simulink model "ev_model_dc7"  (R2020a)
settings: Solver=FixedStepDiscrete  StartTime=0.0  StopTime=20  RelTol=1e-3  EnableMultiTasking=on
PreLoadFcn:
  | assignin('base','Ts',1e-6)
values from neighbouring files (symbols this model uses):
  m = ftell(file)    [calc_coeff.m]    (also in curve_fit_with_error_estimates.m = mean(cp); reheatTest.m = (h6-h5)/(h2-h5))
  s = [s12, s23, s34, s41]    [Rankine.m]    (also in annotation_ifelse.m = subplot(1,2,2); robotic_arm.m = [0]; test_otto.m = plot([0,l2*sind(theta)],             [0,l2*cosd(theta)],    )
undefined symbols (not defined in the file or in its folder): Ion, Lithium
libraries: electricdrivelib x2, powerlib x2, autolibshared x1
settings Model: ExtModeAutoUpdateStatusClock=off  Creator=MathWorks  LastModifiedBy=joshi
settings SolverCC: AutoInsertRateTranBlk=on
settings DataIOCC: LimitDataPoints=on  SaveFormat=Array  SignalLoggingSaveFormat=ModelDataLogs  SaveOutput=off  SignalLogging=off  SaveTime=off  ReturnWorkspaceOutputs=off  SignalLoggingName=sigsOut
settings OptimizationCC: ExpressionDepthLimit=2147483647  InitFltsAndDblsToZero=on  LifeSpan=inf
settings DebuggingCC: UnderspecifiedInitializationDetection=Classic  MergeDetectMultiDrivingBlocksExec=none  CheckExecutionContextPreStartOutputMsg=on  CheckExecutionContextRuntimeOutputMsg=on  SignalResolutionControl=TryResolveAllWithWarning  MultiTaskDSMMsg=warning  MultiTaskCondExecSysMsg=none  FcnCallInpInsideContextMsg=warning  StateNameClashWarn=warning  SFUnexpectedBacktrackingDiag=warning  SFNoUnconditionalDefaultTransitionDiag=warning  SFExecutionAtInitializationDiag=none  ArithmeticOperatorsInVariantConditions=warning
settings HardwareCC: ProdBitPerPointer=32  ProdBitPerSizeT=32  ProdBitPerPtrDiffT=32  ProdLargestAtomicFloat=None  ProdIntDivRoundTo=Undefined  ProdEndianess=Unspecified  ProdWordSize=32  ProdHWDeviceType=32-bit Generic  TargetUnknown=on
settings ModelReferenceCC: PropagateSignalLabelsOutOfModel=off
settings SFSimCC: SimUseLocalCustomCode=off  CustomCodeUndefinedFunction=UseInterfaceOnly
settings RTWCC: RTWUseLocalCustomCode=off
settings CodeAppCC: StateflowObjectComments=on
settings GRTTargetCC: TargetLangStandard=C89/C90 (ANSI)  CombineOutputUpdateFcns=off  GRTInterface=on
settings ConfigComp: CovMetricSettings=dw  CovHtmlReporting=on  CovSaveCumulativeToWorkspaceVar=on  CovSaveSingleToWorkspaceVar=on  CovExternalEMLEnable=off  CovSFcnEnable=off
settings SimscapeCC: SimscapeNormalizeSystem=off

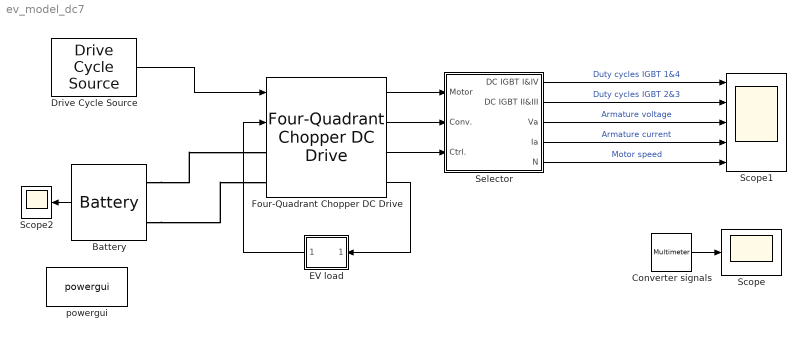
== system ev_model_dc7 ==
  Battery : electricdrivelib/Extra Sources/Battery  BatType=Lithium-Ion  ShowTempParam=off  ThermalPreset=no  ShowAgeParam=off  NomV=352  NomQ=120  SOC=100  Batt_Tr=2  PresetModel=on  MaxQ=120  MinV=264  FullV=409.7235  Dis_rate=52.1739  R=0.029333  Normal_OP=108.5217  expZone="[380.2958      5.895652]"  current=[6.5 13 32.5]  Units=Time  Tci=20  NomT=20  T2=-30  MaxQ2=4.8  FullV2=7.1  Normal_OP2=5.655  expZone2="[6.58           1]"  Rca=0.6  ti=2000  Dp=0  Neq0=0  Tsim=1e6  Ta1=25  Qeol=5.4*0.9  Reol=0.013333*1.2  Char_age=[2.3478, 3]  Dis_age=[2.3478, 10]  N1=1500  N2=10500  N3=1000  N4=1400  Ta2=45  N5=950
  Converter signals : powerlib/Measurements/Multimeter  PhasorSimulation=off  OutputType=Complex  sel=[5 6]  L=10  Gain=[1 1]  yselected={'Uab: Four-Quadrant Chopper DC Drive/Chopper/Chopper/Detailed_4q/IGBT//Diode','Udc: Four-Quadrant Chopper DC Drive/Chopper/Chopper/Detailed_4q/IGBT//Diode'};  PSBOutputType=1  PSBequivalent=0  AxesSetting=[0,0.1,-100,100]  Display=0  SavedBlockNames=-11
      settings: SourceProductBaseCode=MT,PS
  Drive Cycle Source : autolibshared/Drive Cycle Source  cycleVar=.mat, .xls, .xlsx or .txt file  fileVar=D:\MATLAb code files\drive_cycle_ev_dc7.xlsx  tfinal="20  seconds"  cycleRepeat=off  outAccPort=off  outGearPort=off  gearList=No gear data  t_wot1=5  xdot_woto=0  xdot_wot1=30  t_wot2=20  xdot_wot2=0  t_wotend=30  srcUnit=m/s  outUnit=m/s  srcAccUnit=m/s/s  outAccUnit=m/s^2  dt=0.5  aMode=1  faultOption=off  velBnd=2  velBndUnit=mph  inUnit=m/s  timeBnd=1  failOption=off  stopSim=off  maxFaultCnt=10  maxFaultTime=2  maxTotFaultTime=15  traceOption=off  dtTrace=1  traceWindow=10  lastDCname=FTP75 Velocity  lastOutUnit=mph  lastDT=0  lastTB=1  lastSB=2  forceCalcBound=off
      settings: SourceProductBaseCode=PW,MT,VE,VP
  EV load : Subsystem
  Four-Quadrant Chopper DC Drive : electricdrivelib/DC drives/Four-Quadrant Chopper DC Drive  Laf=3.320  Ra=0.076  La=0.00157  Rf=310  Lf=232.25  J=10  Bm=0.32  Tfriction=0  w0=0  smoothingInductance=1e-3  Vfield=310  Ron=1e-3  Vf=1.3  Tf=0  Tt=0  Vfd=1.3  Rsnb=10e3  Csnb=inf  regulationType=Speed regulation  wb=1184  InitialSpeed=0  fc_sc=40  Tsc=100e-6  kp_sc=250  ki_sc=1000  Acc=400  Dec=-400  fc_ic=500  refLim=1.5  switchfreq=5e3  Tic=20e-6  Pb=200*746  Vb=440  kp_ic=2  ki_ic=200  baseSampleTime=1e-06  outputBusMode=Multiple output buses  busLabels=off  MechanicalLoad=Torque Tm  modelDetailLevel=Detailed  driveType=DC7  AverageValue=off
      settings: SourceProductBaseCode=PS
  Scope : Scope
  Scope1 : Scope  NumInputPorts=5
  Scope2 : Scope
  Selector : Subsystem
  powergui : powerlib/powergui  Priority=1  SimulationMode=Discrete  SampleTime=1e-06  frequency=60  Iterations=50  frequencyindice=0  Pbase=100e6  ErrMax=1e-4  UnitsV=kV  UnitsW=MW  buscounter=0  FunctionMessages=off  echomessages=off  EnableUseOfTLC=off  CurrentSourceSwitches=off  DisableSnubberDevices=off  DisableRonSwitches=off  DisableVfSwitches=off  DisplayEquations=off  AutomaticDiscreteSolvers=off  SolverType=Tustin/Backward Euler (TBE)  Interpol=off  ExternalGateDelay=off  methode=off  Ts=100  x0status=blocks  SPID=on  SwTol=0  HookPort=off  NonlinearTolerance=1e-4  nMaxIteration=100  ContinueOnMaxIteration=off  RestoreLinks=warning  ResistiveCurrentMeasurement=off  Frange=[0:2:500]  Ylog=off  Xlog=on  ShowGrid=off  save=off  variable=ZData  structure=0  ZoomFFT=off  StartTime=0.0  cycles=1  DisplayStyle=1  fundamental=60  FreqAxis=off  MaxFrequency=1000  frequencyindicesteady=1  RmsSteady=1  display=off
  wires:
  Selector/1(DC IGBT I&IV) -> Scope1/1  "Duty cycles IGBT 1&4"
  Selector/2(DC IGBT II&III) -> Scope1/2  "Duty cycles IGBT 2&3"
  Selector/3(Va) -> Scope1/3  "Armature voltage"
  Selector/4(Ia) -> Scope1/4  "Armature current"
  Selector/5(N) -> Scope1/5  "Motor speed"
  Converter signals/1 -> Scope/1
  Four-Quadrant Chopper DC Drive/1 -> Selector/1(Motor)
  Four-Quadrant Chopper DC Drive/2 -> Selector/2(Conv.)
  Four-Quadrant Chopper DC Drive/3 -> Selector/3(Ctrl.)
  Drive Cycle Source/1 -> Four-Quadrant Chopper DC Drive/1
  Battery/1 -> Scope2/1
  Four-Quadrant Chopper DC Drive/4 -> EV load/1(In1)
  EV load/1(Out1) -> Four-Quadrant Chopper DC Drive/2
  connections:
  Battery/LConn1 -- Four-Quadrant Chopper DC Drive/LConn1
  Battery/LConn2 -- Four-Quadrant Chopper DC Drive/LConn2

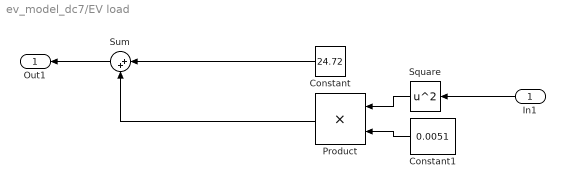
== system ev_model_dc7/EV load ==
  In1 : Inport
  Constant : Constant  Value=24.72
  Constant1 : Constant  Value=0.0051
  Product : Product
  Square : Math  Operator=square  SaturateOnIntegerOverflow=on
  Sum : Sum  Inputs=|++
  Out1 : Outport
  wires:
  Square/1 -> Product/1
  Product/1 -> Sum/2
  Constant1/1 -> Product/2
  Constant/1 -> Sum/1
  Sum/1 -> Out1/1
  In1/1 -> Square/1

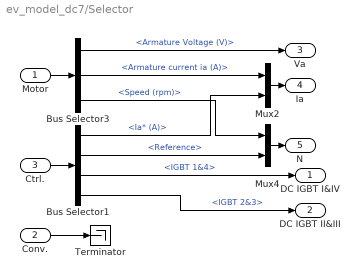
== system ev_model_dc7/Selector ==
  Motor : Inport
  Conv. : Inport  Port=2
  Ctrl. : Inport  Port=3
  Bus Selector1 : BusSelector  OutputSignals=Ia* (A),Reference,Duty Cycles.IGBT 1&4,Duty Cycles.IGBT 2&3
  Bus Selector3 : BusSelector  OutputSignals=Armature Voltage (V),Armature current ia (A),Speed (rpm)
  Mux2 : Mux  Inputs=2
  Mux4 : Mux  Inputs=2
  Terminator : Terminator
  DC IGBT I&IV : Outport  VectorParamsAs1DForOutWhenUnconnected=off
  DC IGBT II&III : Outport  Port=2  VectorParamsAs1DForOutWhenUnconnected=off
  Va : Outport  Port=3  VectorParamsAs1DForOutWhenUnconnected=off
  Ia : Outport  Port=4  VectorParamsAs1DForOutWhenUnconnected=off
  N : Outport  Port=5  VectorParamsAs1DForOutWhenUnconnected=off
  wires:
  Mux2/1 -> Ia/1
  Mux4/1 -> N/1
  Motor/1 -> Bus Selector3/1
  Bus Selector3/1 -> Va/1  "<Armature Voltage (V)>"
  Ctrl./1 -> Bus Selector1/1
  Bus Selector1/1 -> Mux2/2  "<Ia* (A)>"
  Bus Selector1/2 -> Mux4/2  "<Reference>"
  Bus Selector3/2 -> Mux2/1  "<Armature current ia (A)>"
  Bus Selector3/3 -> Mux4/1  "<Speed (rpm)>"
  Conv./1 -> Terminator/1
  Bus Selector1/3 -> DC IGBT I&IV/1  "<IGBT 1&4>"
  Bus Selector1/4 -> DC IGBT II&III/1  "<IGBT 2&3>"
